simulink model "Main_model"  (R2021b)
settings: Solver=ode23t  StartTime=0.0  StopTime=sim_t_end  RelTol=1e-3
undefined symbols (not defined in the file): ambient_co2, ambient_pressure, ambient_rh, ambient_temp, battery, battery_heat_gen_scale, battery_mass, battery_thermal_mass, cab_air_v_dot, cabin_heater_cmd, cabin_heater_max_power, case_cold_plate_mass, case_cold_plate_thermal_mass, chiller_baffles_n, chiller_tube_length, chiller_tubes_n_rows, compressor_max_m_dot, compressor_ref_m_dot, condenser_air_min_flow_area, condenser_tube_width, const_current, coolant_channel_length, coolant_initial_T, coolant_m_dot, coolant_pipe_cross_sec_area, evaporator_air_cross_sec_area, evaporator_air_min_flow_area, evaporator_tube_width, motor_mc_heat_fraction, n_parallel, power_fraction_rear, ptc_heater_max_power, ptc_heater_thermal_mass, rad_air_v_dot, radiator_air_cross_sec_area, radiator_air_min_flow_area, radiator_tube_width, ref_m_dot, ref_pipe_dia, refrigerant_initial_void_fraction, refrigerant_pipe_cross_sec_area, T_bat_active_cool, T_bat_active_heat, T_bat_passive_cool, T_bat_passive_heat, T_battery_init, T_battery_nom, T_cabin_init, T_cabin_setpoint, T_dcdc_nom, T_DT_high, T_DT_passive_cool, T_DT_whr_active, T_front_gb_nom, T_front_mc_nom, T_front_motor_nom, T_rear_gb_nom, T_rear_mc_nom, T_rear_motor_nom, three_w_valve_max_open_area_factor ... (+3)
libraries: fl_lib x448, nesl_utility x328, SimscapeFluids_lib x134, slpidlib x15, ee_lib x9, simulink x8, LiBatteryElements_lib x4, SignalEditorBlockLib x1
(part 23 of 24)

== system Main_model/Battery+DCDC/Battery+DCDC/battery/Charging Algorithm ==
  Constant : Constant  Value=battery.NCell*4.2
  Constant2 : Constant  Value=.85
  Constant5 : Constant  Value=battery.NCell*4.15
  Constant6 : Constant  Value=-const_current
  Delay : Delay  DelayLength=10
  Gain : Gain  Gain=-1
  Gain1 : Gain  Gain=0
  GreaterThan1 : RelationalOperator  Operator=<  OutDataTypeStr=boolean  RndMeth=Simplest
  GreaterThan3 : RelationalOperator  Operator=<  OutDataTypeStr=boolean  RndMeth=Simplest
  NOT : Logic  Operator=NOT  IconShape=distinctive  AllPortsSameDT=off  OutDataTypeStr=boolean
  PID Controller : slpidlib/PID Controller  Controller=PID  Form=Parallel  TimeDomain=Continuous-time  UseExternalTs=off  SampleTime=-1  IntegratorMethod=Forward Euler  FilterMethod=Forward Euler  ControllerParametersSource=internal  P=500  I=0  D=0  UseFilter=on  N=100  TunerSelectOption=Transfer Function Based (PID Tuner App)  InitialConditionSource=internal  InitialConditionForIntegrator=0  InitialConditionForFilter=0  DifferentiatorICPrevScaledInput=0  ExternalReset=none  TrackingMode=off  Kt=1  LimitOutput=on  SatLimitsSource=internal  UpperSaturationLimit=const_current  LowerSaturationLimit=0  LinearizeAsGain=on  AntiWindupMode=none  Kb=1  POutMin=[]  POutMax=[]  IOutMin=[]  IOutMax=[]  DOutMin=[]  DOutMax=[]  NOutMin=[]  NOutMax=[]  SumOutMin=[]  SumOutMax=[]  SaturationOutMin=[]  SaturationOutMax=[]  PParamMin=[]  PParamMax=[]  IParamMin=[]  IParamMax=[]  DParamMin=[]  DParamMax=[]  NParamMin=[]  NParamMax=[]  KbParamMin=[]  KbParamMax=[]  KtParamMin=[]  KtParamMax=[]  KbOutMin=[]  KbOutMax=[]  KtOutMin=[]  KtOutMax=[]  IntegratorOutMin=[]  IntegratorOutMax=[]  FilterOutMin=[]  FilterOutMax=[]  SumI1OutMin=[]  SumI1OutMax=[]  SumI2OutMin=[]  SumI2OutMax=[]  SumI3OutMin=[]  SumI3OutMax=[]  SumI4OutMin=[]  SumI4OutMax=[]  SumDOutMin=[]  SumDOutMax=[]  DifferentiatorOutMin=[]  DifferentiatorOutMax=[]  FilterDiffOutCoefMin=[]  FilterDiffOutCoefMax=[]  ReciprocalOutMin=[]  ReciprocalOutMax=[]  SumDenOutMin=[]  SumDenOutMax=[]  SumNumOutMin=[]  SumNumOutMax=[]  DivideOutMin=[]  DivideOutMax=[]  UdiffTsProdOutMin=[]  UdiffTsProdOutMax=[]  NTsProdOutMin=[]  NTsProdOutMax=[]  UintegralTsProdOutMin=[]  UintegralTsProdOutMax=[]  UngainTsProdOutMin=[]  UngainTsProdOutMax=[]  IntegratorContinuousStateAttributes=''  IntegratorStateMustResolveToSignalObject=off  IntegratorRTWStateStorageClass=Auto  FilterContinuousStateAttributes=''  FilterStateMustResolveToSignalObject=off  FilterRTWStateStorageClass=Auto  ParallelPVariant=InternalParameters  IdealPVariant=Disabled  IVariant=InternalParameters  DVariant=InternalParameters  IntegratorVariant=Continuous  SatVariant=Enabled  AWVariant=Passthrough  PCopyVariant=Disabled  TRVariant=Disabled  FdbkBlocksVariant=Forward  IdealPFdbkVariant=Disabled  SatFdbkVariant=Disabled  DerivativeFilterVariant=ContFilter  NVariant=InternalParameters  NCopyVariant=Disabled  FilterICVariant=InternalICsFilter  IntegratorICVariant=InternalICs  ExternalResetVariant=Disabled  TRSumVariant=Passthrough  SumFdbkVariant=Disabled  SumVariant=Sum_PID  TsampFilterVariant=InternalTs  TsampNgainVariant=Passthrough  TsampIntegralVariant=Passthrough  ExternalSaturationOutDataTypeStr=Inherit: Same as second input
  Scope2 : Scope  NumInputPorts=4
  Scope3 : Scope
  Stop Simulation : Stop
  Sum : Sum  Inputs=|+-
  Switch : Switch  Criteria=u2 > Threshold
  To Workspace : ToWorkspace  VariableName=rear_gb_loss  SaveFormat=Timeseries  SampleTime=-1
  To Workspace1 : ToWorkspace  VariableName=front_gb_loss  SaveFormat=Timeseries  SampleTime=-1
  To Workspace2 : ToWorkspace  VariableName=rear_mc_loss  SaveFormat=Timeseries  SampleTime=-1
  To Workspace3 : ToWorkspace  VariableName=front_mc_loss  SaveFormat=Timeseries  SampleTime=-1
  To Workspace4 : ToWorkspace  VariableName=rear_motor_loss  SaveFormat=Timeseries  SampleTime=-1
  To Workspace5 : ToWorkspace  VariableName=front_motor_loss  SaveFormat=Timeseries  SampleTime=-1
  Transfer Fcn{,3..4,6} (4 alike) : TransferFcn  Denominator=[1 1]
  Transfer Fcn1 : TransferFcn  Denominator=[.1 1]
  Transport Delay2 : TransportDelay  DelayTime=60
  tag scope: bat_I=global, front_gb_heat=global, front_mc_heat=global, front_motor_heat=global, rear_gb_heat=global, rear_mc_heat=global, rear_motor_heat=global
  wires:
  NOT/1 -> Stop Simulation/1
  Gain/1 -> Scope2/2, Switch/3  "PID I output"
  GreaterThan3/1 -> Scope3/1, Switch/2
  Sum/1 -> Scope2/1, PID Controller/1  "PID Input"
  [bat_V] -> Sum/2, Scope2/4, Transfer Fcn6/1  "V_actual"
  Transfer Fcn4/1 -> [bat_I], Scope2/3  "I_actual"
  Transfer Fcn3/1 -> Gain/1
  GreaterThan1/1 -> NOT/1
  Transfer Fcn1/1 -> GreaterThan1/1
  PID Controller/1 -> Transfer Fcn3/1  "PID I output"
  Switch/1 -> Transfer Fcn4/1
  Transfer Fcn6/1 -> GreaterThan3/1
  Constant5/1 -> GreaterThan3/2
  Constant/1 -> Sum/1
  Constant2/1 -> GreaterThan1/2
  Constant6/1 -> Switch/1
  Gain1/1 -> [front_gb_heat], To Workspace1/1, [rear_gb_heat], To Workspace/1, [front_mc_heat], To Workspace3/1, [rear_mc_heat], To Workspace2/1, [front_motor_heat], To Workspace5/1, [rear_motor_heat], To Workspace4/1  "Front GB Heat"
  [soc] -> Transfer Fcn/1, Transfer Fcn1/1
  Transfer Fcn/1 -> Gain1/1

== system Main_model/Battery+DCDC/Battery+DCDC/battery/Elec Battery ==
  note: total_energy_consumed
  ERef : fl_lib/Electrical/Electrical Elements/Electrical Reference
  ERef2 : fl_lib/Electrical/Electrical Elements/Electrical Reference
  Gain : Gain  Gain=1/3600
  Gain1 : Gain  Gain=1/1000
  Gain2 : Gain  Gain=1/3600/1000
  Input Current : fl_lib/Electrical/Electrical Sources/Controlled Current Source
  Integrator : Integrator
  Integrator1 : Integrator
  PS Gain : fl_lib/Physical Signals/Functions/PS Gain  gain=1/n_parallel
  PS-Simulink Converter3 : nesl_utility/PS-Simulink Converter  PhysicalDomain=network_engine_domain  SubClassName=ps_output  LeftPortType=input  RightPortType=output  PseudoPeriodic=off  Frequencies=[]  Unit=inherit  AffineConversion=off
      settings: SourceProductBaseCode=PW,SS
  PS-Simulink Converter4 : nesl_utility/PS-Simulink Converter  PhysicalDomain=network_engine_domain  SubClassName=ps_output  LeftPortType=input  RightPortType=output  PseudoPeriodic=off  Frequencies=[]  Unit=inherit  AffineConversion=off
      settings: SourceProductBaseCode=PW,SS
  PS-Simulink Converter5 : nesl_utility/PS-Simulink Converter  PhysicalDomain=network_engine_domain  SubClassName=ps_output  LeftPortType=input  RightPortType=output  PseudoPeriodic=off  Frequencies=[]  Unit=inherit  AffineConversion=off
      settings: SourceProductBaseCode=PW,SS
  Pack 1 : Subsystem  Tag=PublishSubsystem  mask(Lithium cell (one RC-branch equivalent circuit)){Ncells=battery.NCell, Qe_init=battery.Qe_init, T_init=coolant_initial_T, Capacity_LUT=battery.capacity_LUT, Em_LUT=battery.Em_LUT, R0_LUT=battery.R0_LUT, R1_LUT=battery.R1_LUT, C1_LUT=battery.C1_LUT, cell_mass=battery.cell_mass, cell_Cp_heat=battery.cell_Cp, SOC_LUT=battery.SOC_LUT, Temperature_LUT=battery.temperature_LUT}
      mask prompts: Ncells "Number of series-connected cells"; Qe_init "Initial cell charge deficit (A*hr)"; T_init "Initial cell temperature (K)"; Capacity_LUT "Capacity (A*hr, 1xN table)"; Em_LUT "Em open-circuit voltage, Em (volts, MxN table)"; R0_LUT "R0 terminal resistance (ohms, MxN table)"; R1_LUT "R1 cell resistance (ohms, MxN table)"; C1_LUT "C1 capacitance (farads, MxN table)"; cell_mass "Cell mass (kg)"; cell_Cp_heat "Cell specific heat (J/kg/K)"; SOC_LUT "SOC table breakpoints (Mx1 array)"; Temperature_LUT "Temperature table breakpoints (K, 1xN array)"
      mask DialogControl ParameterTabVar0 Prompt: Main
      mask DialogControl ParameterTabVar01 Prompt: Electrical (per cell)
      mask DialogControl ParameterTabVar012 Prompt: Thermal (per cell)
      mask DialogControl ParameterTabVar0123 Prompt: Table Breakpoints
      mask Display:
      | % Battery icon
      | plot([2.5 1.3],[0 0])
      | plot([-0.6 -1.6 -1.6 -2.5],[0 0 -0.8 -0.8])
      | patch([1 1 -1 -1]*0.15+1.3,[-1 1 1 -1]*0.4,[0;0;0]);
      | patch([1 1 -1 -1]*0.15+0.0,[-1 1 1 -1]*0.4,[0;0;0]);
      | patch([1 1 -1 -1]*0.15+0.7,[-1 1 1 -1]*0.8,[0;0;0]);
      | patch([1 1 -1 -1]*0.15-0.6,[-1 1 1 -1]*0.8,[0;0;0]);
      | % Thermal port
      | plot([-1.6,-1.3],[1.2,1.2])
      | plot([-1.6,-1.3],[0.5,0.5])
      | plot([-1.6,-2.5],[0.8,0.8])
      | plot(0.2*sin(0:2*pi/50:2*pi)-1.6,0.35*cos(0:2*pi/50:2*pi)+0.85)
      | plot(0.2*sin(0:2*pi/50:pi)-1.3,0.35*cos(0:2*pi/50:pi)+0.85)
      | 
      | % Plot points to set plot range
      | color('white');plot(2.5,1.5);plot(-2.5,-1.5)
      | 
      | color('red')
      | port_label('LConn',1,'H')
      | port_label('LConn',2,'+')
      | port_label('RConn',1,'-')
      | port_label('RConn',2,'SOC')
      | port_label('RConn',3,'T')
  Product : Product
  Scope : Scope  NumInputPorts=5
  Simulink-PS Converter1 : nesl_utility/Simulink-PS Converter  PhysicalDomain=network_engine_domain  SubClassName=ps_input  LeftPortType=input  RightPortType=output  PseudoPeriodic=off  Frequencies=[]  NoiseDistribution=none  NoiseParameters=[]  Unit=1  AffineConversion=off  FilteringAndDerivatives=provide  SimscapeFilterOrder=1  InputFilterTimeConstant=0.001  UdotUserProvided=0
      settings: SourceProductBaseCode=PW,SS
  To Workspace1 : ToWorkspace  VariableName=I  SaveFormat=Timeseries  SampleTime=-1
  To Workspace2 : ToWorkspace  VariableName=V  SaveFormat=Timeseries  SampleTime=-1
  To Workspace3 : ToWorkspace  VariableName=battery_heat_gen  SaveFormat=Timeseries  SampleTime=-1
  To Workspace7 : ToWorkspace  VariableName=soc  SaveFormat=Timeseries  SampleTime=-1
  Voltage Sensor : Subsystem
      mask Display: disp('V_load')
  T : PMIOPort  Side=Right
  tag scope: battery_heat=global, soc=global
  wires:
  PS-Simulink Converter4/1 -> Integrator/1, To Workspace3/1, [battery_heat], Scope/2  "heat_gen"
  PS-Simulink Converter3/1 -> To Workspace7/1, [soc], Scope/1  "soc"
  Gain/1 -> Scope/3
  Product/1 -> Integrator1/1, Gain1/1  "pwr"
  Gain2/1 -> Scope/5
  Integrator/1 -> Gain/1  "enery_loss"
  [bat_I] -> To Workspace1/1, Product/1, Simulink-PS Converter1/1
  Integrator1/1 -> Gain2/1
  PS-Simulink Converter5/1 -> To Workspace2/1, Product/2
  Gain1/1 -> Scope/4
  connections:
  Simulink-PS Converter1/RConn1 -- PS Gain/LConn1
  Input Current/RConn2 -- Voltage Sensor/LConn1 -- Pack 1/LConn1
  Pack 1/RConn2 -- PS-Simulink Converter3/LConn1
  Pack 1/RConn4 -- PS-Simulink Converter4/LConn1
  Input Current/LConn1 -- Voltage Sensor/RConn1 -- ERef/LConn1
  ERef2/LConn1 -- Pack 1/RConn1
  PS Gain/RConn1 -- Input Current/RConn1
  PS-Simulink Converter5/LConn1 -- Voltage Sensor/LConn2
  T/RConn1 -- Pack 1/RConn3

== system Main_model/Battery+DCDC/Battery+DCDC/battery/Elec Battery/Pack 1 ==
  note: Scale up voltage drop
      | to total of N cells
  Controlled Voltage Source : fl_lib/Electrical/Electrical Sources/Controlled Voltage Source
  Lithium Cell 1RC : Subsystem  Tag=PublishSubsystem
      mask Display:
      | % Battery icon
      | plot([0 0 0.8 0.8],[0.2 0.9 0.9 1.5])
      | plot([0 0 0.8 0.8],-[0.2 0.9 0.9 1.5])
      | patch([-0.4 0.4 0.4 -0.4],[-0.45 -0.45 -0.15 -0.15],[0;0;0]);
      | patch([-0.9 0.9 0.9 -0.9],[0.15 0.15 0.45 0.45],[0;0;0]);
      | 
      | % Plot points to set plot range
      | color('white');plot(1.5,1.5);plot(-1.5,-1.5)
      | 
      | color('red')
      | port_label('RConn',1,'P')
      | port_label('RConn',2,'+')
      | port_label('LConn',1,'T')
      | port_label('LConn',2,'-')
  N : fl_lib/Physical Signals/Functions/PS Gain  gain=Ncells*n_parallel
  N-1 : fl_lib/Physical Signals/Functions/PS Gain  gain=(Ncells-1)
  Voltage Sensor : fl_lib/Electrical/Electrical Sensors/Voltage Sensor
  - : PMIOPort  Tag=PMCPort  Side=Right
  + : PMIOPort  Tag=PMCPort  Port=2  Side=Left
  SOC : PMIOPort  Port=3  Side=Right
  T : PMIOPort  Port=4  Side=Right
  heat_gen : PMIOPort  Port=5  Side=Right
  connections:
  SOC/RConn1 -- Lithium Cell 1RC/RConn2
  N/LConn1 -- Lithium Cell 1RC/RConn1
  T/RConn1 -- Lithium Cell 1RC/LConn1
  heat_gen/RConn1 -- N/RConn1
  Controlled Voltage Source/LConn1 -- Voltage Sensor/RConn2 -- Lithium Cell 1RC/LConn2
  N-1/LConn1 -- Voltage Sensor/RConn1
  Voltage Sensor/LConn1 -- Lithium Cell 1RC/RConn3 -- +/RConn1
  N-1/RConn1 -- Controlled Voltage Source/RConn1
  Controlled Voltage Source/RConn2 -- -/RConn1

== system Main_model/Battery+DCDC/Battery+DCDC/battery/Elec Battery/Voltage Sensor ==
  PS-Simulink Converter : nesl_utility/PS-Simulink Converter  PhysicalDomain=network_engine_domain  SubClassName=ps_output  LeftPortType=input  RightPortType=output  PseudoPeriodic=off  Frequencies=[]  Unit=inherit  AffineConversion=off
      settings: SourceProductBaseCode=PW,SS
  Voltage Sensor : fl_lib/Electrical/Electrical Sensors/Voltage Sensor
  + : PMIOPort  Side=Left
  - : PMIOPort  Port=2  Side=Right
  Connection Port : PMIOPort  Port=3  Side=Left
  tag scope: bat_V=global
  wires:
  PS-Simulink Converter/1 -> [bat_V]
  connections:
  -/RConn1 -- Voltage Sensor/RConn2
  +/RConn1 -- Voltage Sensor/LConn1
  Voltage Sensor/RConn1 -- PS-Simulink Converter/LConn1 -- Connection Port/RConn1

== system Main_model/Battery+DCDC/Battery+DCDC/battery/Elec Battery/Pack 1/Lithium Cell 1RC ==
  note: Power
      | Losses
  C1 : LiBatteryElements_lib/C_table  C_Table=C1_LUT F  SOC_Table=SOC_LUT  Temp_Table=Temperature_LUT K  v0=0 V
      settings: SourceProductBaseCode=SS  InternalSimscapePortConfiguration="{\"Bottom\":[],\"Left\":[{\"id\":\"p\",\"label\":\"+\",\"type\":\"foundation.electrical.electrical\"},{\"id\":\"T\",\"label\":\"T\",\"type\":\"input\"},{\"id\":\"SOC\",\"label\":\"SOC\",\"type\":\"input\"}],\"Right\":[{\"id\":\"n\",\"label\":\"-\",\"type\":\"foundation.electrical.electrical\"}],\"Top\":[]}"
  Em_table : LiBatteryElements_lib/Em_table  C_Table=Capacity_LUT hr*A  Em_Table=Em_LUT V  SOC_Table=SOC_LUT  Temp_Table=Temperature_LUT K  Qinit=Qe_init hr*A
      settings: SourceProductBaseCode=SS  InternalSimscapePortConfiguration="{\"Bottom\":[],\"Left\":[{\"id\":\"p\",\"label\":\"+\",\"type\":\"foundation.electrical.electrical\"},{\"id\":\"C\",\"label\":\"C\",\"type\":\"output\"},{\"id\":\"SOC\",\"label\":\"SOC\",\"type\":\"output\"}],\"Right\":[{\"id\":\"n\",\"label\":\"-\",\"type\":\"foundation.electrical.electrical\"},{\"id\":\"T\",\"label\":\"T\",\"type\":\"input\"}],\"Top\":[]}"
  PS Add : fl_lib/Physical Signals/Functions/PS Add
  PS Constant : fl_lib/Physical Signals/Sources/PS Constant  constant=25
  PS Constant1 : fl_lib/Physical Signals/Sources/PS Constant  constant=.1
  R0 : LiBatteryElements_lib/R_table  R_Table=R0_LUT Ohm  SOC_Table=SOC_LUT  Temp_Table=Temperature_LUT K
      settings: SourceProductBaseCode=SS  InternalSimscapePortConfiguration="{\"Bottom\":[],\"Left\":[{\"id\":\"p\",\"label\":\"+\",\"type\":\"foundation.electrical.electrical\"},{\"id\":\"T\",\"label\":\"T\",\"type\":\"input\"},{\"id\":\"SOC\",\"label\":\"SOC\",\"type\":\"input\"}],\"Right\":[{\"id\":\"n\",\"label\":\"-\",\"type\":\"foundation.electrical.electrical\"},{\"id\":\"pow\",\"label\":\"POW\",\"type\":\"output\"}],\"Top\":[]}"
  R1 : LiBatteryElements_lib/R_table  R_Table=R1_LUT Ohm  SOC_Table=SOC_LUT  Temp_Table=Temperature_LUT K
      settings: SourceProductBaseCode=SS  InternalSimscapePortConfiguration="{\"Bottom\":[],\"Left\":[{\"id\":\"p\",\"label\":\"+\",\"type\":\"foundation.electrical.electrical\"},{\"id\":\"T\",\"label\":\"T\",\"type\":\"input\"},{\"id\":\"SOC\",\"label\":\"SOC\",\"type\":\"input\"}],\"Right\":[{\"id\":\"n\",\"label\":\"-\",\"type\":\"foundation.electrical.electrical\"},{\"id\":\"pow\",\"label\":\"POW\",\"type\":\"output\"}],\"Top\":[]}"
  P : PMIOPort  Side=Right
  T : PMIOPort  Port=2  Side=Left
  SOC : PMIOPort  Port=3  Side=Right
  + : PMIOPort  Port=4  Side=Right
  - : PMIOPort  Port=5  Side=Left
  connections:
  C1/LConn3 -- R0/LConn3 -- SOC/RConn1 -- Em_table/LConn3 -- R1/LConn3
  Em_table/RConn1 -- -/RConn1
  R0/LConn1 -- R1/RConn1 -- C1/RConn1
  PS Add/LConn2 -- R0/RConn2
  PS Add/LConn1 -- R1/RConn2
  R1/LConn1 -- C1/LConn1 -- Em_table/LConn1
  R1/LConn2 -- C1/LConn2 -- R0/LConn2 -- T/RConn1 -- Em_table/RConn2
  +/RConn1 -- R0/RConn1
  PS Add/RConn1 -- P/RConn1

== matlab function Main_model/HP Control Systems Ideal WHR (+ Summer modes) /Valves Control ==
  data: v1 output; v2 output; v3 output; v4 output; v5 output; v6 output; v7 output; v8 output; v9 output; v10 output; T_cabin input; T_amb input; T_battery input; T_DT_max input; current_mode output; T_DT_min input; T_bat_passive_cool parameter; T_DT_whr_active parameter; T_bat_active_cool parameter; T_bat_passive_heat parameter; T_bat_active_heat parameter; T_DT_passive_cool parameter; T_DT_high parameter; T_cabin_setpoint parameter
function [v1,v2,v3,v4,v5,v6,v7,v8,v9,v10,current_mode]= fcn(T_cabin, T_amb, T_battery, T_DT_max, T_DT_min,T_bat_passive_cool, T_DT_whr_active, T_bat_active_cool, T_bat_passive_heat, T_bat_active_heat, T_DT_passive_cool, T_DT_high,T_cabin_setpoint)

if T_amb<T_cabin_setpoint-273
    if T_battery<T_bat_passive_heat
        if T_battery<T_bat_active_heat
            if T_DT_min<T_DT_whr_active
                mode(1)
            elseif T_DT_max<T_DT_high  
                mode(2)
            else
                mode(2.25)
            end
        else
            if T_DT_min<T_DT_whr_active
                mode(1)
            elseif T_DT_max<T_DT_high
                mode(2.5)
            else
                mode(2.75)
            end
        end
    elseif T_battery >=T_bat_passive_heat && T_battery<T_bat_passive_cool
        if T_DT_min<T_DT_whr_active
            mode(5)
        elseif T_DT_max<T_DT_high
            mode(6)
        else
            mode(6.25)   
        end
    else
        if T_battery>=T_bat_passive_cool && T_battery<=T_bat_active_cool
            if T_DT_min<T_DT_whr_active
                mode(4)
            elseif T_DT_max<T_DT_high
                mode(3)
            else
                mode(3.25)    
            end            
        else
            if T_DT_min<T_DT_whr_active
                mode(4.25)
            elseif T_DT_max<T_DT_high
                mode(3.5)
            else 
                mode(3.75)
            end                            
        end
    end

else
    if T_battery<=T_bat_passive_cool
        if T_DT_max<=T_DT_passive_cool
            mode(9)
        else
            mode(9.25)
        end        
    else
        if T_battery>=T_bat_passive_cool && T_battery<=T_bat_active_cool
            if T_DT_max<=T_DT_passive_cool
                mode(8)
            else
                mode(7)
            end            
        else
            if T_DT_max<=T_DT_passive_cool
                mode(8.25)
            else
                mode(7.25)
            end 
        end        
    end

end

% mode(11)

    function reset_valves()
        v1=0;
        v2=0;
        v3=0;
        v4=0;
        v5=0;
        v6=0;
        v7=0;
        v8=0;
        v9=0;
        v10=0;
    end
    function mode(x)
        reset_valves()
        if x==1
            v2=1;
            v3=1;
            v6=1;
            current_mode=1;
        elseif x==2 
            v3=1;
            v6=1;
            v5=1;
            current_mode=2;
        elseif x==2.25        
            v3=1;
            v6=1;
            v5=1;
            v10=1;
            current_mode=2.25;            
        elseif x==2.5
            v2=1;
            v3=1;
            v8=1;
            current_mode=2.5;
        elseif x==2.75
            v2=1;
            v3=1;
            v8=1;
            v10=1;
            current_mode=2.75;            
        elseif x==3
            v3=1;
            if T_battery<T_DT_min
                v5=1;
            else
                v7=1;
            end
            current_mode=3;
        elseif x==3.25
            v3=1;
            v10=1;
            if T_battery<T_DT_min
                v5=1;
            else
                v7=1;
            end
            current_mode=3.25;        
        elseif x==3.5
            v3=1;
            v9=1;
            if T_battery<T_DT_min
                v5=1;
            else
                v7=1;
            end            
            current_mode=3.5;
        elseif x==3.75
            v3=1;
            v9=1;
            v10=1;            
            if T_battery<T_DT_min
                v5=1;
            else
                v7=1;
            end
            current_mode=3.75;            
        elseif x==4
            v3=1;
            v7=1;            
            current_mode=4;
        elseif x==4.25
            v3=1;
            v7=1;
            v9=1;            
            current_mode=4.25;
        elseif x==5
            v2=1;
            v3=1;            
            current_mode=5;
        elseif x==6
            v3=1;
            v5=1;            
            current_mode=6;
        elseif x==6.25
            v3=1;
            v5=1;
            v10=1;            
            current_mode=6.25;
%         elseif x==7 || x==7.25
%             v2=1;
%             v6=1;                        
%             current_mode=7;

        elseif x==7
            v1=1;
            v4=1;
            v9=1;            
            v10=1;            
            current_mode=7;
        elseif x==7.25
            v1=1;
            v4=1;
            v7=1;            
            v10=1;            
            current_mode=7.25;
        elseif x==8
            v1=1;
            v4=1;
            v9=1;
            current_mode=8;
        elseif x==8.25
            v1=1;
            v4=1;
            v7=1;            
            current_mode=8.25;
        elseif x==9
            v1=1;
            v4=1;            
            current_mode=9;
        elseif x==9.25
            v1=1;
            v4=1;           
            v10=1;            
            current_mode=9.25;
        else
            error('Mode not Valid')
        end
    end
end

== matlab function Main_model/Compressor/Refrigerant Mass Flow Rate Controls /MATLAB Function4 ==
  data: in input; out output; time input
function out = fcn(in, time)
    if time>500
        a=.1;
        b=.2;
        x= (in-a)/(b-a);
        if x<0
            out=0;
        elseif x>1
            out=1;
        else
    %         out=3*x^2-2*x^3;
            out=6*x^5-15*x^4+10*x^3;
        end
    else
        out=1;
    end

end

== matlab function Main_model/HP Control Systems Battery to Chiller WHR /Valves Control ==
  data: v1 output; v2 output; v3 output; v4 output; v5 output; v6 output; v7 output; v8 output; v9 output; v10 output; T_cabin input; T_amb input; T_battery input; T_DT_max input; T_DT_min input; current_mode output; T_bat_passive_cool parameter; T_bat_passive_heat parameter; T_bat_active_cool parameter; T_DT_passive_cool parameter; T_cabin_setpoint parameter
function [v1,v2,v3,v4,v5,v6,v7,v8,v9,v10,current_mode]= fcn(T_cabin, T_amb, T_battery, T_DT_max, T_DT_min, T_bat_passive_cool, T_bat_passive_heat, T_bat_active_cool, T_DT_passive_cool,T_cabin_setpoint)

if T_amb<T_cabin_setpoint-273
    if T_battery<T_bat_passive_heat
        if T_DT_max<T_DT_passive_cool
            mode(1)
        else 
            mode(2)
        end
    elseif T_battery >=T_bat_passive_heat && T_battery<=T_bat_passive_cool
        if T_DT_max<T_DT_passive_cool
            mode(3)
        else 
            mode(4)
        end
    elseif T_battery <T_bat_active_cool
        if T_DT_max<T_DT_passive_cool
            mode(5)
        else 
            mode(6)
        end
    else 
        if T_DT_max<T_DT_passive_cool
            mode(5.25)
        else 
            mode(6.25)
        end        
    end

elseif T_amb >=17 && T_cabin<=23
    if T_battery<T_bat_passive_cool
        if T_DT_max<=T_DT_passive_cool
            mode(10)
        else
            mode(10.25)
        end
    else
        if T_battery>=T_bat_passive_cool && T_battery<=T_bat_active_cool
            if T_DT_max<=T_DT_passive_cool
                mode(9)
            else
                mode(8)
            end            
        else
            if T_DT_max<=T_DT_passive_cool
                mode(9.25)
            else
                mode(8.25)
            end 
        end
    end

else
    if T_battery<=T_bat_passive_cool
        if T_DT_max<=T_DT_passive_cool
            mode(13)
        else
            mode(13.25)
        end        
    else
        if T_battery>=T_bat_passive_cool && T_battery<=T_bat_active_cool
            if T_DT_max<=T_DT_passive_cool
                mode(12)
            else
                mode(11)
            end            
        else
            if T_DT_max<=T_DT_passive_cool
                mode(12.25)
            else
                mode(11.25)
            end 
        end        
    end

end

    function reset_valves()
        v1=0;
        v2=0;
        v3=0;
        v4=0;
        v5=0;
        v6=0;
        v7=0;
        v8=0;
        v9=0;
        v10=0;
    end
    function mode(x)
        reset_valves()
        if x==1
            v2=1;
            v3=1;
            v6=1;
            current_mode=1;
        elseif x==2
            v2=1;
            v3=1;
            v6=1;
            v10=1;
            current_mode=2;          
        elseif x==3
            v2=1;
            v3=1;
            current_mode=3;           
        elseif x==4
            v2=1;
            v3=1; 
            v10=1;
            current_mode=4;
        elseif x==5
            v3=1;
            v7=1;
            current_mode=5;
        elseif x==5.25
            v3=1;
            v7=1;
            v9=1;
            current_mode=5.25;            
        elseif x==6
            v3=1;
            v7=1;
            v10=1;
            current_mode=6;
        elseif x==6.25
            v3=1;
            v7=1;
            v9=1;
            v10=1;
            current_mode=6.25;            
        elseif x==7
            v2=1;
            v6=1;                        
            current_mode=7;
        elseif x==8
            v9=1;
            v10=1;                        
            current_mode=8;
        elseif x==8.25
            v1=1;
            v7=1;              
            v10=1;              
            current_mode=8.25;
        elseif x==9
            v9=1;              
            current_mode=9;
        elseif x==9.25
            v1=1;
            v7=1;              
            current_mode=9.25;
        elseif x==10              
            current_mode=10;
        elseif x==10.25
            v10=1;            
            current_mode=10.25;
        elseif x==11
            v1=1;
            v4=1;
            v9=1;            
            v10=1;            
            current_mode=11;
        elseif x==11.25
            v1=1;
            v4=1;
            v7=1;            
            v10=1;            
            current_mode=11.25;
        elseif x==12
            v1=1;
            v4=1;            
            current_mode=12;
        elseif x==12.25
            v1=1;
            v4=1;
            v7=1;            
            current_mode=12.25;
        elseif x==13
            v1=1;
            v4=1;            
            current_mode=13;
        elseif x==13.25
            v1=1;
            v4=1;           
            v10=1;            
            current_mode=13.25;
        else
            error('Mode not Valid')
        end
    end
end

== matlab function Main_model/HP Control Systems DT to Battery WHR /Valves Control ==
  data: v1 output; v2 output; v3 output; v4 output; v5 output; v6 output; v7 output; v8 output; v9 output; v10 output; T_cabin input; T_amb input; T_battery input; T_DT_max input; T_DT_min input; current_mode output; T_bat_passive_cool parameter; T_DT_whr_active parameter; T_bat_active_cool parameter; T_bat_passive_heat parameter; T_bat_active_heat parameter; T_DT_passive_cool parameter; T_DT_high parameter; T_cabin_setpoint parameter
function [v1,v2,v3,v4,v5,v6,v7,v8,v9,v10,current_mode]= fcn(T_cabin, T_amb, T_battery, T_DT_max, T_DT_min,T_bat_passive_cool, T_DT_whr_active, T_bat_active_cool, T_bat_passive_heat, T_bat_active_heat, T_DT_passive_cool, T_DT_high,T_cabin_setpoint)

if T_amb<T_cabin_setpoint-273
    if T_battery<T_bat_passive_heat
        if T_battery<T_bat_active_heat
            if T_DT_min<T_DT_whr_active
                mode(1)
            else 
                mode(2)
            end
        else
            if T_DT_min<T_DT_whr_active
                mode(1)
            elseif T_DT_max<T_DT_high
                mode(2.25)   
            else
                mode(2.5)
            end
        end       
    elseif T_battery >=T_bat_passive_heat && T_battery<=T_bat_passive_cool
        if T_DT_max<T_DT_passive_cool
            mode(3)
        else 
            mode(4)
        end
    else
        if T_DT_max<T_DT_passive_cool
            mode(5)
        else 
            mode(6)
        end
    end

elseif T_amb >=17 && T_cabin<=23
    if T_battery<T_bat_passive_cool
        if T_DT_max<=T_DT_passive_cool
            mode(10)
        else
            mode(10.25)
        end
    else
        if T_battery>=T_bat_passive_cool && T_battery<=T_bat_active_cool
            if T_DT_max<=T_DT_passive_cool
                mode(9)
            else
                mode(8)
            end            
        else
            if T_DT_max<=T_DT_passive_cool
                mode(9.25)
            else
                mode(8.25)
            end 
        end
    end

else
    if T_battery<=T_bat_passive_cool
        if T_DT_max<=T_DT_passive_cool
            mode(13)
        else
            mode(13.25)
        end        
    else
        if T_battery>=T_bat_passive_cool && T_battery<=T_bat_active_cool
            if T_DT_max<=T_DT_passive_cool
                mode(12)
            else
                mode(11)
            end            
        else
            if T_DT_max<=T_DT_passive_cool
                mode(12.25)
            else
                mode(11.25)
            end 
        end        
    end

end

    function reset_valves()
        v1=0;
        v2=0;
        v3=0;
        v4=0;
        v5=0;
        v6=0;
        v7=0;
        v8=0;
        v9=0;
        v10=0;
    end
    function mode(x)
        reset_valves()
        if x==1
            v2=1;
            v3=1;
            v6=1;
            current_mode=1;
        elseif x==2
            v2=1;
            v3=1;
            v6=1;
            v10=1;
            current_mode=2;
        elseif x==2.25
            v2=1;
            v3=1;
            v8=1;
            current_mode=2.25;
        elseif x==2.5
            v2=1;
            v3=1;
            v8=1;
            v10=1;
            current_mode=2.5;         
        elseif x==3
            v2=1;
            v3=1;
            current_mode=3;           
        elseif x==4
            v2=1;
            v3=1; 
            v10=1;
            current_mode=4;
        elseif x==5
            v2=1;
            v3=1;
            v9=1;
            current_mode=5;
        elseif x==6
            v2=1;
            v3=1;
            v9=1;
            v10=1;
            current_mode=6;
        elseif x==7
            v2=1;
            v6=1;                        
            current_mode=7;
        elseif x==8
            v9=1;
            v10=1;                        
            current_mode=8;
        elseif x==8.25
            v1=1;
            v7=1;              
            v10=1;              
            current_mode=8.25;
        elseif x==9
            v9=1;              
            current_mode=9;
        elseif x==9.25
            v1=1;
            v7=1;              
            current_mode=9.25;
        elseif x==10              
            current_mode=10;
        elseif x==10.25
            v10=1;            
            current_mode=10.25;
        elseif x==11
            v1=1;
            v4=1;
            v9=1;            
            v10=1;            
            current_mode=11;
        elseif x==11.25
            v1=1;
            v4=1;
            v7=1;            
            v10=1;            
            current_mode=11.25;
        elseif x==12
            v1=1;
            v4=1;            
            current_mode=12;
        elseif x==12.25
            v1=1;
            v4=1;
            v7=1;            
            current_mode=12.25;
        elseif x==13
            v1=1;
            v4=1;            
            current_mode=13;
        elseif x==13.25
            v1=1;
            v4=1;           
            v10=1;            
            current_mode=13.25;
        else
            error('Mode not Valid')
        end
    end
end

== matlab function Main_model/Compressor/Refrigerant Mass Flow Rate Controls /MATLAB Function ==
  data: current_mode input; comp_off output
function comp_off = fcn(current_mode)
if current_mode==7 || current_mode==8 || current_mode==9 || current_mode==10 || current_mode==10.25
    comp_off=0;
else 
    comp_off=1;
end
end

== matlab function Main_model/Compressor/Refrigerant Mass Flow Rate Controls /MATLAB Function1 ==
  data: in input; out output
function out = fcn(in)
    a=.08;%.1; %0.08;
    b=.15;%.2; %0.15;
    x= (in-a)/(b-a);
    if x<0
        out=0;
    elseif x>1
        out=1;
    else
%         out=3*x^2-2*x^3;
        out=6*x^5-15*x^4+10*x^3;
    end

end

== matlab function Main_model/HVAC cycles/compressor4/Refrigerant Mass Flow Rate Controls /MATLAB Function ==
  data: current_mode input; comp_off output
function comp_off = fcn(current_mode)
if current_mode==7 || current_mode==8 || current_mode==9 || current_mode==10 || current_mode==10.25
    comp_off=0;
else 
    comp_off=1;
end
end

== matlab function Main_model/HVAC cycles/compressor4/Refrigerant Mass Flow Rate Controls /MATLAB Function1 ==
  data: in input; out output
function out = fcn(in)
    a=.08;%.1; %0.08;
    b=.15;%.2; %0.15;
    x= (in-a)/(b-a);
    if x<0
        out=0;
    elseif x>1
        out=1;
    else
%         out=3*x^2-2*x^3;
        out=6*x^5-15*x^4+10*x^3;
    end

end

== matlab function Main_model/HVAC cycles/compressor4/Refrigerant Mass Flow Rate Controls /MATLAB Function2 ==
  data: in input; out output
function out = fcn(in)
    a=2;   %2
    b=2.5; %2.75
    x= (in-a)/(b-a);
    if x<0
        out=1;
    elseif x>1
        out=0;
    else
%         out=3*x^2-2*x^3;
        out=1-(6*x^5-15*x^4+10*x^3);
    end

end

== matlab function Main_model/HVAC cycles/compressor1/Refrigerant Mass Flow Rate Controls /MATLAB Function2 ==
  data: in input; out output
function out = fcn(in)
    a=2;   %2
    b=2.5; %2.75
    x= (in-a)/(b-a);
    if x<0
        out=1;
    elseif x>1
        out=0;
    else
%         out=3*x^2-2*x^3;
        out=1-(6*x^5-15*x^4+10*x^3);
    end

end

== matlab function Main_model/Compressor/Refrigerant Mass Flow Rate Controls /MATLAB Function2 ==
  data: in input; out output
function out = fcn(in)
    a=2;   %2
    b=2.5; %2.75
    x= (in-a)/(b-a);
    if x<0
        out=1;
    elseif x>1
        out=0;
    else
%         out=3*x^2-2*x^3;
        out=1-(6*x^5-15*x^4+10*x^3);
    end

end

== matlab function Main_model/PTC Control Systems (Follow steps inside for PTC analysis)/Valves Control ==
  data: v1 output; v2 output; v3 output; v4 output; v5 output; v6 output; v7 output; v8 output; v9 output; v10 output; ptc_heater output; T_cabin input; T_amb input; T_battery input; T_DT_max input; current_mode output; T_DT_min input; T_bat_passive_heat parameter; T_bat_passive_cool parameter; T_DT_passive_cool parameter; T_bat_active_cool parameter; T_cabin_setpoint parameter
function [v1,v2,v3,v4,v5,v6,v7,v8,v9,v10,ptc_heater, current_mode]= fcn(T_cabin, T_amb, T_battery, T_DT_max, T_DT_min, T_bat_passive_heat, T_bat_passive_cool, T_DT_passive_cool, T_bat_active_cool,T_cabin_setpoint)

if T_amb<T_cabin_setpoint-273
    if T_battery<T_bat_passive_heat
        if T_DT_max<T_DT_passive_cool
            mode(1)
        else 
            mode(2)
        end
    elseif T_battery >=T_bat_passive_heat && T_battery<=T_bat_passive_cool
        if T_DT_max<T_DT_passive_cool
            mode(3)
        else 
            mode(4)
        end
    else
        if T_DT_max<T_DT_passive_cool
            mode(5)
        else 
            mode(6)
        end
    end

elseif T_amb >=17 && T_cabin<=23
    if T_battery<T_bat_passive_cool
        if T_DT_max<=T_DT_passive_cool
            mode(10)
        else
            mode(10.25)
        end
    else
        if T_battery>=T_bat_passive_cool && T_battery<=T_bat_active_cool
            if T_DT_max<=T_DT_passive_cool
                mode(9)
            else
                mode(8)
            end            
        else
            if T_DT_max<=T_DT_passive_cool
                mode(9.25)
            else
                mode(8.25)
            end 
        end
    end

else
    if T_battery<=T_bat_passive_cool
        if T_DT_max<=T_DT_passive_cool
            mode(13)
        else
            mode(13.25)
        end        
    else
        if T_battery>=T_bat_passive_cool && T_battery<=T_bat_active_cool
            if T_DT_max<=T_DT_passive_cool
                mode(12)
            else
                mode(11)
            end            
        else
            if T_DT_max<=T_DT_passive_cool
                mode(12.25)
            else
                mode(11.25)
            end 
        end        
    end

end

    function reset_valves()
        v1=0;
        v2=0;
        v3=0;
        v4=0;
        v5=0;
        v6=0;
        v7=0;
        v8=0;
        v9=0;
        v10=0;
        ptc_heater=0;
    end
    function mode(x)
        reset_valves()
        if x==1
            v3=1;
            v6=1;
            ptc_heater=1;
            current_mode=1;
        elseif x==2
            v3=1;
            v6=1;
            v10=1;
            ptc_heater=1;
            current_mode=2;          
        elseif x==3
            v3=1;
            ptc_heater=1;
            current_mode=3;           
        elseif x==4
            v3=1; 
            v10=1;
            ptc_heater=1;
            current_mode=4;
        elseif x==5
            v3=1;
            v9=1;
            ptc_heater=1;
            current_mode=5;
        elseif x==6
            v3=1;
            v9=1;
            v10=1;
            ptc_heater=1;
            current_mode=6;
        elseif x==7
            v2=1;
            v6=1;                        
            current_mode=7;
        elseif x==8
            v9=1;
            v10=1;                        
            current_mode=8;
        elseif x==8.25
            v1=1;
            v7=1;              
            v10=1;              
            current_mode=8.25;
        elseif x==9
            v9=1;              
            current_mode=9;
        elseif x==9.25
            v1=1;
            v7=1;              
            current_mode=9.25;
        elseif x==10              
            current_mode=10;
        elseif x==10.25
            v10=1;            
            current_mode=10.25;
        elseif x==11
            v1=1;
            v4=1;
            v9=1;            
            v10=1;            
            current_mode=11;
        elseif x==11.25
            v1=1;
            v4=1;
            v7=1;            
            v10=1;            
            current_mode=11.25;
        elseif x==12
            v1=1;
            v4=1;            
            current_mode=12;
        elseif x==12.25
            v1=1;
            v4=1;
            v7=1;            
            current_mode=12.25;
        elseif x==13
            v1=1;
            v4=1;            
            current_mode=13;
        elseif x==13.25
            v1=1;
            v4=1;           
            v10=1;            
            current_mode=13.25;
        else
            error('Mode not Valid')
        end
    end
end

== matlab function Main_model/HVAC cycles/compressor4/Refrigerant Mass Flow Rate Controls /MATLAB Function3 ==
  data: in input; out output
function out = fcn(in)
    comp_power_scale=1;
    a=comp_power_scale*1.8;   %2
    b=comp_power_scale*2; %2.75
    x= (in-a)/(b-a);
    if x<0
        out=1;
    elseif x>1
        out=0;
    else
%         out=3*x^2-2*x^3;
        out=1-(6*x^5-15*x^4+10*x^3);
    end

end

== matlab function Main_model/HVAC cycles/compressor1/Refrigerant Mass Flow Rate Controls /MATLAB Function3 ==
  data: in input; out output
function out = fcn(in)
    comp_power_scale=1;
    a=comp_power_scale*1.8;   %2
    b=comp_power_scale*2; %2.75
    x= (in-a)/(b-a);
    if x<0
        out=1;
    elseif x>1
        out=0;
    else
%         out=3*x^2-2*x^3;
        out=1-(6*x^5-15*x^4+10*x^3);
    end

end

== matlab function Main_model/Compressor/Refrigerant Mass Flow Rate Controls /MATLAB Function3 ==
  data: in input; out output
function out = fcn(in)
    comp_power_scale=2;
    b=comp_power_scale*2+0.15;
    a=b-0.1;  
    x= (in-a)/(b-a);
    if x<0
        out=1;
    elseif x>1
        out=0;
    else
%         out=3*x^2-2*x^3;
        out=1-(6*x^5-15*x^4+10*x^3);
    end

end

== matlab function Main_model/HP Control Systems No WHR/Valves Control ==
  data: v1 output; v2 output; v3 output; v4 output; v5 output; v6 output; v7 output; v8 output; v9 output; v10 output; T_cabin input; T_amb input; T_battery input; T_DT_max input; current_mode output; T_DT_min input; T_bat_passive_heat parameter; T_bat_passive_cool parameter; T_DT_passive_cool parameter; T_bat_active_cool parameter; T_cabin_setpoint parameter
function [v1,v2,v3,v4,v5,v6,v7,v8,v9,v10,current_mode]= fcn(T_cabin, T_amb, T_battery, T_DT_max, T_DT_min, T_bat_passive_heat, T_bat_passive_cool, T_DT_passive_cool, T_bat_active_cool,T_cabin_setpoint)

if T_amb<T_cabin_setpoint-273
    if T_battery<T_bat_passive_heat
        if T_DT_max<T_DT_passive_cool
            mode(1)
        else 
            mode(2)
        end
    elseif T_battery >=T_bat_passive_heat && T_battery<=T_bat_passive_cool
        if T_DT_max<T_DT_passive_cool
            mode(3)
        else 
            mode(4)
        end
    else
        if T_DT_max<T_DT_passive_cool
            mode(5)
        else 
            mode(6)
        end
    end

elseif T_amb >=17 && T_cabin<=23
    if T_battery<T_bat_passive_cool
        if T_DT_max<=T_DT_passive_cool
            mode(10)
        else
            mode(10.25)
        end
    else
        if T_battery>=T_bat_passive_cool && T_battery<=T_bat_active_cool
            if T_DT_max<=T_DT_passive_cool
                mode(9)
            else
                mode(8)
            end            
        else
            if T_DT_max<=T_DT_passive_cool
                mode(9.25)
            else
                mode(8.25)
            end 
        end
    end

else
    if T_battery<=T_bat_passive_cool
        if T_DT_max<=T_DT_passive_cool
            mode(13)
        else
            mode(13.25)
        end        
    else
        if T_battery>=T_bat_passive_cool && T_battery<=T_bat_active_cool
            if T_DT_max<=T_DT_passive_cool
                mode(12)
            else
                mode(11)
            end            
        else
            if T_DT_max<=T_DT_passive_cool
                mode(12.25)
            else
                mode(11.25)
            end 
        end        
    end

end

    function reset_valves()
        v1=0;
        v2=0;
        v3=0;
        v4=0;
        v5=0;
        v6=0;
        v7=0;
        v8=0;
        v9=0;
        v10=0;
    end
    function mode(x)
        reset_valves()
        if x==1
            v2=1;
            v3=1;
            v6=1;
            current_mode=1;
        elseif x==2
            v2=1;
            v3=1;
            v6=1;
            v10=1;
            current_mode=2;          
        elseif x==3
            v2=1;
            v3=1;
            current_mode=3;           
        elseif x==4
            v2=1;
            v3=1; 
            v10=1;
            current_mode=4;
        elseif x==5
            v2=1;
            v3=1;
            v9=1;
            current_mode=5;
        elseif x==6
            v2=1;
            v3=1;
            v9=1;
            v10=1;
            current_mode=6;
        elseif x==7
            v2=1;
            v6=1;                        
            current_mode=7;
        elseif x==8
            v9=1;
            v10=1;                        
            current_mode=8;
        elseif x==8.25
            v1=1;
            v7=1;              
            v10=1;              
            current_mode=8.25;
        elseif x==9
            v9=1;              
            current_mode=9;
        elseif x==9.25
            v1=1;
            v7=1;              
            current_mode=9.25;
        elseif x==10              
            current_mode=10;
        elseif x==10.25
            v10=1;            
            current_mode=10.25;
        elseif x==11
            v1=1;
            v4=1;
            v9=1;            
            v10=1;            
            current_mode=11;
        elseif x==11.25
            v1=1;
            v4=1;
            v7=1;            
            v10=1;            
            current_mode=11.25;
        elseif x==12
            v1=1;
            v4=1;            
            current_mode=12;
        elseif x==12.25
            v1=1;
            v4=1;
            v7=1;            
            current_mode=12.25;
        elseif x==13
            v1=1;
            v4=1;            
            current_mode=13;
        elseif x==13.25
            v1=1;
            v4=1;           
            v10=1;            
            current_mode=13.25;
        else
            error('Mode not Valid')
        end
    end
end

== matlab function Main_model/Components Library/Compressor/Refrigerant Mass Flow Rate Controls /MATLAB Function ==
  data: current_mode input; comp_off output
function comp_off = fcn(current_mode)
if current_mode==7 || current_mode==8 || current_mode==9 || current_mode==10 || current_mode==10.25
    comp_off=0;
else 
    comp_off=1;
end
end

== matlab function Main_model/Components Library/Compressor/Refrigerant Mass Flow Rate Controls /MATLAB Function1 ==
  data: in input; out output
function out = fcn(in)
    a=.08;%.1; %0.08;
    b=.15;%.2; %0.15;
    x= (in-a)/(b-a);
    if x<0
        out=0;
    elseif x>1
        out=1;
    else
%         out=3*x^2-2*x^3;
        out=6*x^5-15*x^4+10*x^3;
    end

end

== matlab function Main_model/Components Library/Compressor/Refrigerant Mass Flow Rate Controls /MATLAB Function2 ==
  data: in input; out output
function out = fcn(in)
    a=2;   %2
    b=2.5; %2.75
    x= (in-a)/(b-a);
    if x<0
        out=1;
    elseif x>1
        out=0;
    else
%         out=3*x^2-2*x^3;
        out=1-(6*x^5-15*x^4+10*x^3);
    end

end

== matlab function Main_model/Components Library/Compressor/Refrigerant Mass Flow Rate Controls /MATLAB Function3 ==
  data: in input; out output
function out = fcn(in)
    comp_power_scale=2;
    b=comp_power_scale*2+0.15;
    a=b-0.1;  
    x= (in-a)/(b-a);
    if x<0
        out=1;
    elseif x>1
        out=0;
    else
%         out=3*x^2-2*x^3;
        out=1-(6*x^5-15*x^4+10*x^3);
    end

end

== matlab function Main_model/Components Library/Compressor/Refrigerant Mass Flow Rate Controls /MATLAB Function4 ==
  data: in input; out output; time input
function out = fcn(in, time)
    if time>500
        a=.1;
        b=.2;
        x= (in-a)/(b-a);
        if x<0
            out=0;
        elseif x>1
            out=1;
        else
    %         out=3*x^2-2*x^3;
            out=6*x^5-15*x^4+10*x^3;
        end
    else
        out=1;
    end

end

== matlab function Main_model/HVAC cycles/compressor1/Refrigerant Mass Flow Rate Controls /MATLAB Function ==
  data: current_mode input; comp_off output
function comp_off = fcn(current_mode)
if current_mode==7 || current_mode==8 || current_mode==9 || current_mode==10 || current_mode==10.25
    comp_off=0;
else 
    comp_off=1;
end
end

== matlab function Main_model/HVAC cycles/compressor1/Refrigerant Mass Flow Rate Controls /MATLAB Function1 ==
  data: in input; out output
function out = fcn(in)
    a=.08;%.1; %0.08;
    b=.15;%.2; %0.15;
    x= (in-a)/(b-a);
    if x<0
        out=0;
    elseif x>1
        out=1;
    else
%         out=3*x^2-2*x^3;
        out=6*x^5-15*x^4+10*x^3;
    end

end
